simulink model "task_3"  (R2017b)
settings: Solver=VariableStepAuto  StartTime=0.0  StopTime=1000  RelTol=1e-3
values from neighbouring files (symbols this model uses):
  g = 9.81    [task_3.m]    (also in task_3_e.m)
  k_d_phi = (2*seta_phi*omega_phi - a_1)/a_2    [task_3_e.m]
  k_i_chi = (omega_chi^2)*V_a/g    [task_3_e.m]
  k_p_chi = 2*seta_chi*omega_chi*V_a/g    [task_3_e.m]
  k_p_phi = -(u_max/e_max)    (= -2)    [task_3_e.m]
  V_a = 580    [task_1_all.m]    (also in task_3.m = 161.111111111; task_3_e.m = 161.111111111)
libraries: simulink x2
settings Model: Creator=Ivan  LastModifiedBy=Ivan

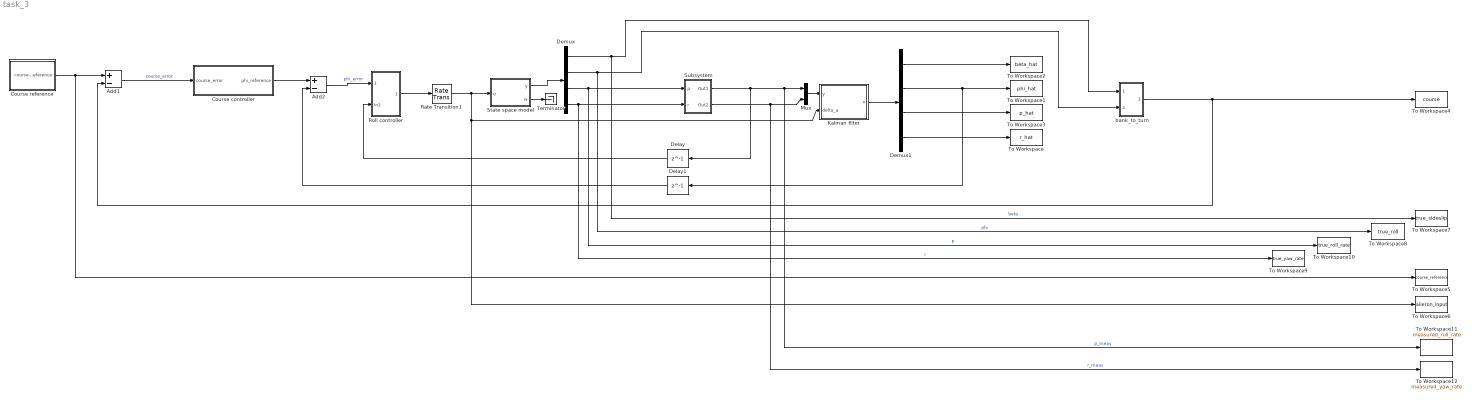
== system task_3 ==
  Add1 : Sum  Inputs=+-
  Add2 : Sum  Inputs=+-
  Course controller : Subsystem
  Course reference : Subsystem
  Delay : Delay  DelayLength=1  InitialCondition=0
  Delay1 : Delay  DelayLength=1  InitialCondition=0
  Demux : Demux
  Demux1 : Demux
  Kalman filter : MATLAB Function  TreatAsAtomicUnit=on
  Mux : Mux  Inputs=2
  Rate Transition1 : RateTransition  OutPortSampleTime=0.01
  Roll controller : Subsystem
  State space model : MATLAB Function  TreatAsAtomicUnit=on
  Subsystem : Subsystem
  Terminator : Terminator
  To Workspace : ToWorkspace  VariableName=r_hat  SaveFormat=Structure With Time  SampleTime=-1
  To Workspace1 : ToWorkspace  VariableName=phi_hat  SaveFormat=Structure With Time  SampleTime=-1
  To Workspace10 : ToWorkspace  VariableName=true_roll_rate  SaveFormat=Structure With Time  SampleTime=-1
  To Workspace11 : ToWorkspace  VariableName=measured_roll_rate  SaveFormat=Structure With Time  SampleTime=-1
  To Workspace12 : ToWorkspace  VariableName=measured_yaw_rate  SaveFormat=Structure With Time  SampleTime=-1
  To Workspace2 : ToWorkspace  VariableName=beta_hat  SaveFormat=Structure With Time  SampleTime=-1
  To Workspace3 : ToWorkspace  VariableName=p_hat  SaveFormat=Structure With Time  SampleTime=-1
  To Workspace4 : ToWorkspace  VariableName=course  SaveFormat=Structure With Time  SampleTime=-1
  To Workspace5 : ToWorkspace  VariableName=course_reference  SaveFormat=Structure With Time  SampleTime=-1
  To Workspace6 : ToWorkspace  VariableName=aileron_input  SaveFormat=Structure With Time  SampleTime=-1
  To Workspace7 : ToWorkspace  VariableName=true_sideslip  SaveFormat=Structure With Time  SampleTime=-1
  To Workspace8 : ToWorkspace  VariableName=true_roll  SaveFormat=Structure With Time  SampleTime=-1
  To Workspace9 : ToWorkspace  VariableName=true_yaw_rate  SaveFormat=Structure With Time  SampleTime=-1
  bank_to_turn : Subsystem
  wires:
  Course reference/1(course reference) -> To Workspace5/1, Add1/1
  Add1/1 -> Course controller/1(course_error)  "course_error"
  Course controller/1(phi_reference) -> Add2/1
  Add2/1 -> Roll controller/1(phi_error)  "phi_error"
  Roll controller/1(delta_a) -> Rate Transition1/1
  Rate Transition1/1 -> To Workspace6/1, Kalman filter/2(delta_a), State space model/1(u)
  State space model/2(w) -> Terminator/1
  State space model/1(y) -> Demux/1
  Demux/3 -> To Workspace10/1, Subsystem/1(p)  "p"
  Demux/4 -> To Workspace9/1, Subsystem/2(r)  "r"
  Subsystem/1(Out1) -> Delay/1, To Workspace11/1, Mux/1  "p_meas"
  Subsystem/2(Out2) -> To Workspace12/1, Mux/2  "r_meas"
  Mux/1 -> Kalman filter/1(y)
  Kalman filter/1(x) -> Demux1/1
  Demux1/1 -> To Workspace2/1
  Demux1/2 -> To Workspace1/1, Delay1/1
  Demux1/3 -> To Workspace3/1
  Demux1/4 -> To Workspace/1
  Delay/1 -> Roll controller/2(In2)
  Delay1/1 -> Add2/2
  Demux/1 -> To Workspace7/1, bank_to_turn/1(beta)  "beta"
  Demux/2 -> To Workspace8/1, bank_to_turn/2(phi)  "phi"
  bank_to_turn/1(course) -> Add1/2, To Workspace4/1

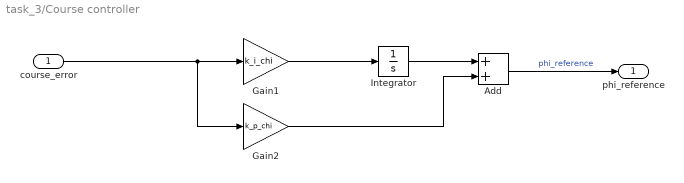
== system task_3/Course controller ==
  course_error : Inport
  Add : Sum
  Gain1 : Gain  Gain=k_i_chi
  Gain2 : Gain  Gain=k_p_chi
  Integrator : Integrator
  phi_reference : Outport
  wires:
  Integrator/1 -> Add/1
  Gain1/1 -> Integrator/1
  Add/1 -> phi_reference/1  "phi_reference"
  course_error/1 -> Gain2/1, Gain1/1
  Gain2/1 -> Add/2

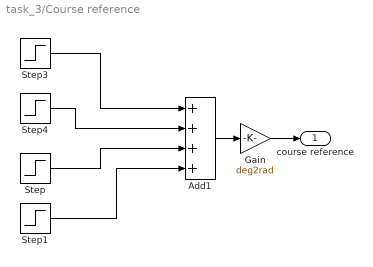
== system task_3/Course reference ==
  Add1 : Sum  Inputs=++++
  Gain : Gain  Gain=deg2rad
  Step : Step  Time=625  After=-5  SampleTime=0
  Step1 : Step  Time=750  After=-5  SampleTime=0
  Step3 : Step  Time=250  After=15  SampleTime=0
  Step4 : Step  Time=500  After=-5  SampleTime=0
  course reference : Outport
  wires:
  Step4/1 -> Add1/2
  Step1/1 -> Add1/4
  Step/1 -> Add1/3
  Add1/1 -> Gain/1
  Step3/1 -> Add1/1
  Gain/1 -> course reference/1

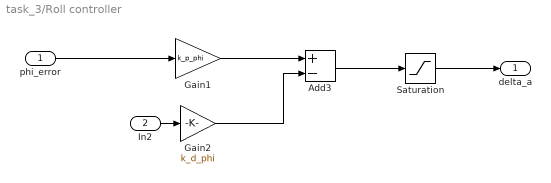
== system task_3/Roll controller ==
  phi_error : Inport
  In2 : Inport  Port=2
  Add3 : Sum  Inputs=+-
  Gain1 : Gain  Gain=k_p_phi
  Gain2 : Gain  Gain=k_d_phi
  Saturation : Saturate  UpperLimit=30*deg2rad  LowerLimit=-30*deg2rad
  delta_a : Outport
  wires:
  Gain2/1 -> Add3/2
  Add3/1 -> Saturation/1
  In2/1 -> Gain2/1
  phi_error/1 -> Gain1/1
  Gain1/1 -> Add3/1
  Saturation/1 -> delta_a/1

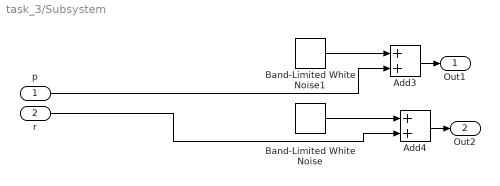
== system task_3/Subsystem ==
  p : Inport
  r : Inport  Port=2
  Add3 : Sum
  Add4 : Sum
  Band-Limited White Noise : simulink/Sources/Band-Limited White Noise  Cov=[(0.2*deg2rad)^2]  Ts=0.01  seed=[23358]
  Band-Limited White Noise1 : simulink/Sources/Band-Limited White Noise  Cov=[(0.2*deg2rad)^2]  Ts=0.01  seed=[23341]
  Out1 : Outport
  Out2 : Outport  Port=2
  wires:
  p/1 -> Add3/2
  r/1 -> Add4/2
  Add4/1 -> Out2/1
  Add3/1 -> Out1/1
  Band-Limited White Noise1/1 -> Add3/1
  Band-Limited White Noise/1 -> Add4/1

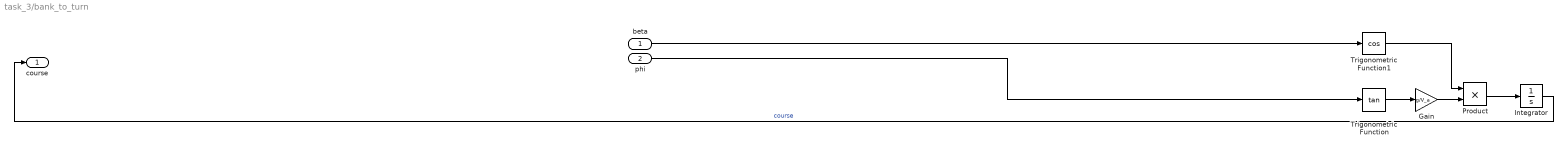
== system task_3/bank_to_turn ==
  beta : Inport
  phi : Inport  Port=2
  Gain : Gain  Gain=g/V_a
  Integrator : Integrator
  Product : Product
  Trigonometric Function : Trigonometry  Operator=tan
  Trigonometric Function1 : Trigonometry  Operator=cos
  course : Outport
  wires:
  beta/1 -> Trigonometric Function1/1
  phi/1 -> Trigonometric Function/1
  Trigonometric Function1/1 -> Product/1
  Integrator/1 -> course/1  "course"
  Gain/1 -> Product/2
  Trigonometric Function/1 -> Gain/1
  Product/1 -> Integrator/1

== matlab function task_3/Kalman filter ==
  data: y input; x output; delta_a input
function x = kf(y, delta_a)
    P_0 = 10^-5*diag([0.001 1 100 10]);
    x_0 = zeros(4, 1);
    x = kalman_filter(y, delta_a, P_0, x_0);
end

== matlab function task_3/State space model ==
  data: u input; y output; w output
function [y, w] = ss(u)
    [y, w] = state_space_example(u);
end
